simulink model "PROJEKT_SM"  (R2019b)
settings: Solver=FixedStepAuto  StartTime=0.0  StopTime=8000  FixedStep=1  RelTol=1e-3
libraries: simulink x1
settings Model: Creator=wilin  LastModifiedBy=wilin

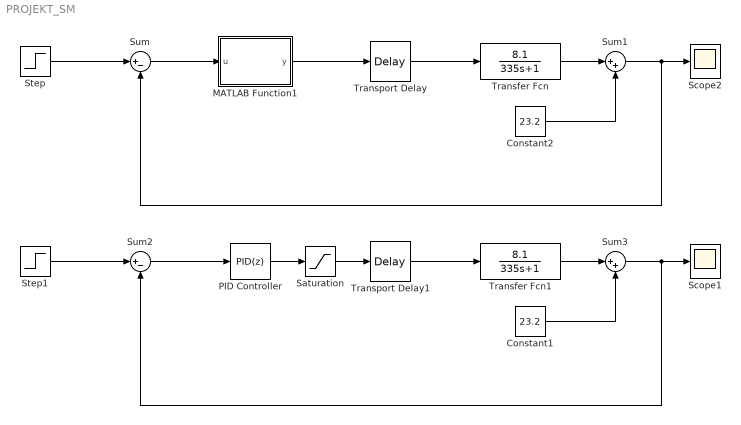
== system PROJEKT_SM ==
  Constant1 : Constant  Value=23.2
  Constant2 : Constant  Value=23.2
  MATLAB Function1 : MATLAB Function  TreatAsAtomicUnit=on
  PID Controller : simulink/Continuous/PID Controller  Controller=PID  Form=Parallel  TimeDomain=Discrete-time  SampleTime=1  IntegratorMethod=Forward Euler  FilterMethod=Forward Euler  ControllerParametersSource=internal  P=1  I=0.005  D=0.4  UseFilter=off  N=100  TunerSelectOption=Transfer Function Based (PID Tuner App)  InitialConditionSource=internal  InitialConditionForIntegrator=0  InitialConditionForFilter=0  DifferentiatorICPrevScaledInput=0  ExternalReset=none  TrackingMode=off  Kt=1  LimitOutput=off  UpperSaturationLimit=inf  LowerSaturationLimit=-inf  LinearizeAsGain=on  AntiWindupMode=none  Kb=1  POutMin=[]  POutMax=[]  IOutMin=[]  IOutMax=[]  DOutMin=[]  DOutMax=[]  NOutMin=[]  NOutMax=[]  SumOutMin=[]  SumOutMax=[]  SaturationOutMin=[]  SaturationOutMax=[]  PParamMin=[]  PParamMax=[]  IParamMin=[]  IParamMax=[]  DParamMin=[]  DParamMax=[]  NParamMin=[]  NParamMax=[]  KbParamMin=[]  KbParamMax=[]  KtParamMin=[]  KtParamMax=[]  KbOutMin=[]  KbOutMax=[]  KtOutMin=[]  KtOutMax=[]  IntegratorOutMin=[]  IntegratorOutMax=[]  FilterOutMin=[]  FilterOutMax=[]  SumI1OutMin=[]  SumI1OutMax=[]  SumI2OutMin=[]  SumI2OutMax=[]  SumI3OutMin=[]  SumI3OutMax=[]  SumI4OutMin=[]  SumI4OutMax=[]  SumDOutMin=[]  SumDOutMax=[]  DifferentiatorOutMin=[]  DifferentiatorOutMax=[]  FilterDiffOutCoefMin=[]  FilterDiffOutCoefMax=[]  ReciprocalOutMin=[]  ReciprocalOutMax=[]  SumDenOutMin=[]  SumDenOutMax=[]  SumNumOutMin=[]  SumNumOutMax=[]  DivideOutMin=[]  DivideOutMax=[]  IntegratorContinuousStateAttributes=''  IntegratorStateMustResolveToSignalObject=off  IntegratorRTWStateStorageClass=Auto  FilterContinuousStateAttributes=''  FilterStateMustResolveToSignalObject=off  FilterRTWStateStorageClass=Auto  ParallelPVariant=InternalParameters  IdealPVariant=Disabled  IVariant=InternalParameters  DVariant=InternalParameters  IntegratorVariant=Discrete  SatVariant=Disabled  AWVariant=Passthrough  PCopyVariant=Disabled  TRVariant=Disabled  FdbkBlocksVariant=Forward  IdealPFdbkVariant=Disabled  SatFdbkVariant=Disabled  DerivativeFilterVariant=Differentiator  NVariant=Passthrough  NCopyVariant=Disabled_SignalSpec  FilterICVariant=InternalICsDifferentiator  IntegratorICVariant=InternalICs  ExternalResetVariant=Disabled  TRSumVariant=Passthrough  SumFdbkVariant=Disabled  SumVariant=Sum_PID
  Saturation : Saturate  UpperLimit=1  LowerLimit=0
  Scope1 : Scope
  Scope2 : Scope
  Step : Step  Time=0  After=26  SampleTime=0
  Step1 : Step  Time=0  After=26  SampleTime=0
  Sum : Sum  Inputs=|+-
  Sum1 : Sum  Inputs=|++
  Sum2 : Sum  Inputs=|+-
  Sum3 : Sum  Inputs=|++
  Transfer Fcn : TransferFcn  Numerator=[8.1]  Denominator=[335 1]
  Transfer Fcn1 : TransferFcn  Numerator=[8.1]  Denominator=[335 1]
  Transport Delay : TransportDelay  DelayTime=10
  Transport Delay1 : TransportDelay  DelayTime=10
  wires:
  Step/1 -> Sum/1
  Sum/1 -> MATLAB Function1/1(u)
  MATLAB Function1/1(y) -> Transport Delay/1
  Transport Delay/1 -> Transfer Fcn/1
  Transfer Fcn/1 -> Sum1/1
  Sum1/1 -> Sum/2, Scope2/1
  Constant2/1 -> Sum1/2
  Sum2/1 -> PID Controller/1
  Step1/1 -> Sum2/1
  Sum3/1 -> Sum2/2, Scope1/1
  Transport Delay1/1 -> Transfer Fcn1/1
  Constant1/1 -> Sum3/2
  Transfer Fcn1/1 -> Sum3/1
  PID Controller/1 -> Saturation/1
  Saturation/1 -> Transport Delay1/1

== matlab function PROJEKT_SM/MATLAB Function1 ==
  settings: updateMethod=DISCRETE  sampleTime=1
  data: u input; y output
function y = PID(u)

    Kp = 20.45;
    Ki = 0.222;
    Kd = 470.35;
    
    persistent prev_error
    if isempty(prev_error)
        prev_error = 0;
    end
     
    persistent prev_int
    if isempty(prev_int)
        prev_int = 0;
    end
    
    persistent prev_anti
    if isempty(prev_anti)
        prev_anti = 0;
    end
    
    error = u;
    
    integral = prev_int + ((error + (0 * prev_anti)) + prev_error);
    prev_int = integral;
    
    deriv = (error - prev_error)/1;
    prev_error = error;
    
    ster = Kp*error + Ki*integral * (1.0/2.0) + Kd*deriv;
    
    if ster > 1
        prev_anti = 1 - ster;
        ster = 1;
    elseif ster < 0
        prev_anti = 0 - ster;
        ster = 0;
    else
        prev_anti = 0;
    end
    
    y = ster;
